simulink model "eq_2_6_model"  (R2025a)
settings: Solver=VariableStepAuto  StartTime=0.0  StopTime=100  RelTol=1e-3
values from neighbouring files (symbols this model uses):
  a = linspace(0.01, 5, 200)    [b26_e1.m]    (also in b26_e3.m; ic26.m = 1; iic26.m = 1; iiic26.m = 1)
  b = linspace(-5, 5, 200)    [b26_e1.m]    (also in b26_e3.m = linspace(-3, 3, 200); ic26.m = 1; iic26.m = -0.5; iiic26.m = -2)
  x10 = 0    [ic26.m]    (also in iic26.m; iiic26.m)
  x20 = 0    [ic26.m]    (also in iic26.m; iiic26.m)
settings Model: Creator=Nenad  LastModifiedBy=Korisnik

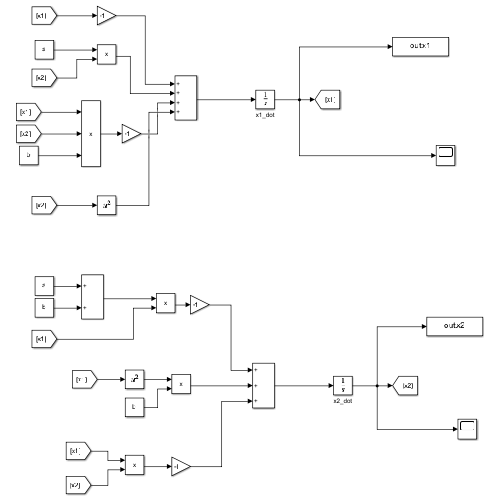
[thumbnail: Simulink's stored preview of the top-level diagram]
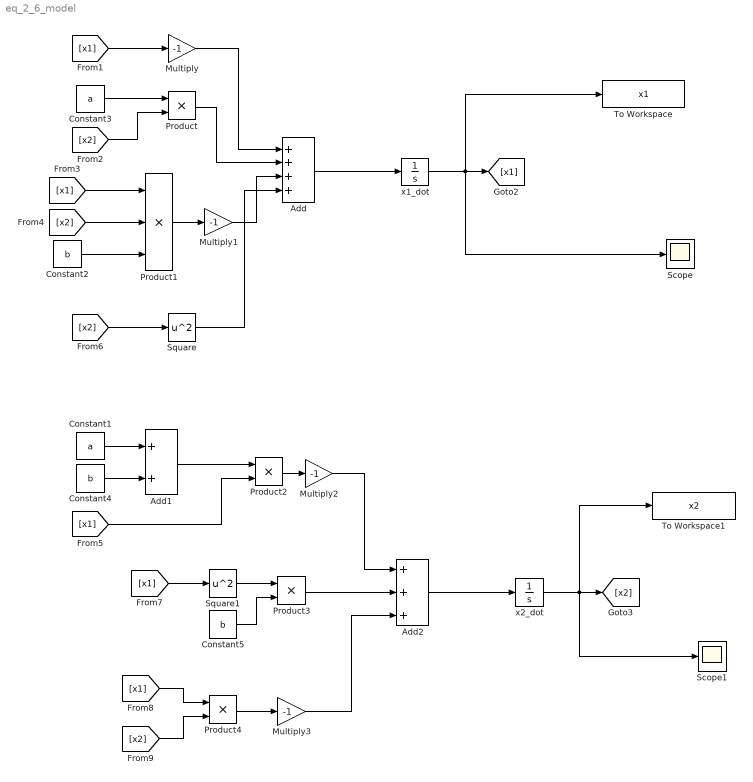
== system eq_2_6_model ==
  Add : Sum  Inputs=4
  Add1 : Sum
  Add2 : Sum  Inputs=3
  Constant1 : Constant  Value=a
  Constant2 : Constant  Value=b
  Constant3 : Constant  Value=a
  Constant4 : Constant  Value=b
  Constant5 : Constant  Value=b
  Multiply{,1..3} (4 alike) : Gain  Gain=-1
  Product{,2..4} (4 alike) : Product
  Product1 : Product  Inputs=3
  Scope : Scope
      settings: ActiveDisplayYMinimum=-1  ActiveDisplayYMaximum=1
  Scope1 : Scope
      settings: ActiveDisplayYMinimum=-1.592419478775521  ActiveDisplayYMaximum=-0.73420920077439289
  Square : Math  Operator=square
  Square1 : Math  Operator=square
  To Workspace : ToWorkspace  VariableName=x1  SaveFormat=Timeseries  SampleTime=-1
  To Workspace1 : ToWorkspace  VariableName=x2  SaveFormat=Timeseries  SampleTime=-1
  x1_dot : Integrator  InitialCondition=x10
  x2_dot : Integrator  InitialCondition=x20
  wires:
  x1_dot/1 -> Scope/1, To Workspace/1, [x1]
  x2_dot/1 -> Scope1/1, To Workspace1/1, [x2]
  [x1] -> Multiply/1
  Constant3/1 -> Product/1
  [x2] -> Product/2
  [x1] -> Product1/1
  [x2] -> Product1/2
  [x2] -> Square/1
  Multiply/1 -> Add/1
  Product/1 -> Add/2
  Add/1 -> x1_dot/1
  Constant1/1 -> Add1/1
  Constant4/1 -> Add1/2
  [x1] -> Product2/2
  [x1] -> Square1/1
  Square1/1 -> Product3/1
  Constant5/1 -> Product3/2
  [x1] -> Product4/1
  [x2] -> Product4/2
  Product3/1 -> Add2/2
  Add2/1 -> x2_dot/1
  Product4/1 -> Multiply3/1
  Multiply3/1 -> Add2/3
  Add1/1 -> Product2/1
  Product2/1 -> Multiply2/1
  Multiply2/1 -> Add2/1
  Constant2/1 -> Product1/3
  Product1/1 -> Multiply1/1
  Multiply1/1 -> Add/3
  Square/1 -> Add/4
